simulink model "drone"  (R2020b)
settings: Solver=VariableStepAuto  StartTime=0.0  StopTime=10.0  RelTol=1e-3
settings Model: Creator=91869  LastModifiedBy=91869

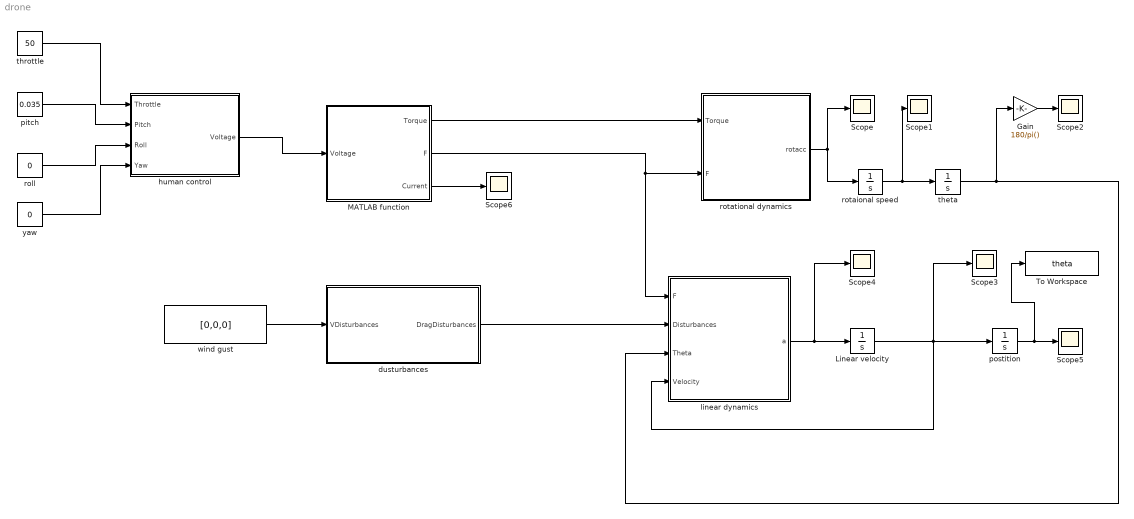
== system drone ==
  Gain : Gain  Gain=180/pi()
  Linear velocity : Integrator
  MATLAB function : MATLAB Function  TreatAsAtomicUnit=on
  Scope{,1..6} (7 alike) : Scope
  To Workspace : ToWorkspace  VariableName=theta  SampleTime=-1
      settings: Save2DSignal=2-D array (concatenate along first dimension)
  dusturbances : MATLAB Function  TreatAsAtomicUnit=on
  human control : MATLAB Function  TreatAsAtomicUnit=on
  linear dynamics : MATLAB Function  TreatAsAtomicUnit=on
  pitch : Constant  Value=0.035
  postition : Integrator
  roll : Constant  Value=0
  rotaional speed : Integrator
  rotational dynamics : MATLAB Function  TreatAsAtomicUnit=on
  theta : Integrator
  throttle : Constant  Value=50
  wind gust : Constant  Value=[0,0,0]
  yaw : Constant  Value=0
  wires:
  MATLAB function/2(F) -> linear dynamics/1(F), rotational dynamics/2(F)
  MATLAB function/1(Torque) -> rotational dynamics/1(Torque)
  rotational dynamics/1(rotacc) -> rotaional speed/1, Scope/1
  rotaional speed/1 -> Scope1/1, theta/1
  theta/1 -> Gain/1, linear dynamics/3(Theta)
  linear dynamics/1(a) -> Scope4/1, Linear velocity/1
  Linear velocity/1 -> Scope3/1, linear dynamics/4(Velocity), postition/1
  dusturbances/1(DragDisturbances) -> linear dynamics/2(Disturbances)
  wind gust/1 -> dusturbances/1(VDisturbances)
  yaw/1 -> human control/4(Yaw)
  roll/1 -> human control/3(Roll)
  pitch/1 -> human control/2(Pitch)
  throttle/1 -> human control/1(Throttle)
  human control/1(Voltage) -> MATLAB function/1(Voltage)
  postition/1 -> To Workspace/1, Scope5/1
  Gain/1 -> Scope2/1
  MATLAB function/3(Current) -> Scope6/1

== matlab function drone/rotational dynamics ==
  data: Torque input; rotacc output; F input
function rotacc = fcn(Torque,F)
Moment=[0 0 0];
rotacc=[0 0 0];
I=[0.003,0.003,0.007];
Moment(1)=(F(3)+F(4))*0.237/2-(F(1)+F(2))*0.237/2;
Moment(2)=(F(3)+F(2))*0.237/2-(F(1)+F(4))*0.237/2;
Moment(3)=Torque(4)-Torque(1)+Torque(2)-Torque(3);
for i=1:3
    rotacc(i)=Moment(i)/I(i);
end

== matlab function drone/MATLAB function ==
  data: Voltage input; Torque output; F output; Current output
function [Torque,F,Current]=fcn(Voltage)
RPM=[0 0 0 0];
Torque=[0 0 0 0];
Current=[0 0 0 0];
F=[0 0 0 0];
for i=1:4
    RPM(i)=-2.6931*Voltage(i)^3+1400*Voltage(i);
    Ct=2*10^-15*RPM(i)^3-4*10^-11*RPM(i)^2+3*10^-7*RPM(i)+0.1013;
    F(i)=Ct*1.225*(RPM(i)/60)^2*0.2^4;
    Torque(i)=4*10^-14*RPM(i)^3+8*10^-12*RPM(i)^2+3*10^-6*RPM(i);
    Current(i)=1400*Torque(i);
end

== matlab function drone/linear dynamics ==
  data: F input; a output; Disturbances input; Theta input; Velocity input
function a = fcn(F,Disturbances,Theta,Velocity)
m=0.743;
g=9.81;
A=[0.0197,0.0197,0.0512];
rho=1.225;
Cd=1;

a=[0 0 0];
Force=[0 0 0];
Fprop=[0 0 0];

Fprop(1)=sin(Theta(2))*cos(Theta(1))*(F(1)+F(2)+F(3)+F(4));
Fprop(2)=sin(Theta(1))*cos(Theta(2))*(F(1)+F(2)+F(3)+F(4));
Fprop(3)=cos(Theta(2))*cos(Theta(1))*(F(1)+F(2)+F(3)+F(4));

ThetaXY=-atan2(Fprop(1),Fprop(2));
XY2D=sqrt(Fprop(1)^2+Fprop(2)^2);

if Fprop(3)>=0
    Fprop(1)=XY2D*sin(ThetaXY+Theta(3));
    Fprop(2)=XY2D*cos(ThetaXY+Theta(3));
else
    Fprop(1)=XY2D*sin(-ThetaXY+Theta(3));
    Fprop(2)=XY2D*cos(-ThetaXY+Theta(3));
end
if Velocity(1)<0
    Force(1)=Fprop(1)-Disturbances(1)+0.5*rho*Velocity(1)^2*A(1)*Cd;
else
    Force(1)=Fprop(1)-Disturbances(1)-0.5*rho*Velocity(1)^2*A(1)*Cd;
end    
if Velocity(2)<0
    Force(2)=Fprop(2)-Disturbances(2)+0.5*rho*Velocity(2)^2*A(2)*Cd;
else
    Force(2)=Fprop(2)-Disturbances(2)-0.5*rho*Velocity(2)^2*A(2)*Cd;
end
if Velocity(3)<0
    Force(3)=Fprop(3)-Disturbances(3)+0.5*rho*Velocity(3)^2*A(3)*Cd-m*g;
else
    Force(3)=Fprop(3)-Disturbances(3)-0.5*rho*Velocity(3)^2*A(3)*Cd-m*g;
end

for i=1:3
    a(i)=Force(i)/m;
end

== matlab function drone/dusturbances ==
  data: VDisturbances input; DragDisturbances output
function DragDisturbances = fcn(VDisturbances)
A=[0.0197 0.0197 0.0197*2*1.3];
rho=1.225;
Cd=1;
DragDisturbances=[0 0 0];

for i=1:3
    if VDisturbances(i)<0
        DragDisturbances(i)=0.5*rho*VDisturbances(i)^2*A(i)*Cd;
    else    
        DragDisturbances(i)=-0.5*rho*VDisturbances(i)^2*A(i)*Cd;
    end
end

== matlab function drone/human control ==
  data: Throttle input; Voltage output; Pitch input; Roll input; Yaw input
function Voltage = fcn(Throttle,Pitch,Roll,Yaw)
Correct=0;
if (Pitch/2+Roll/2+Yaw/2)>(100-Throttle)
    Correct=(Pitch/2+Roll/2+Yaw/2)-(100-Throttle); 
end

if (Pitch/2+Roll/2+Yaw)>(Throttle-10)
    if Correct<(Pitch/2+Yaw/2+Roll/2)-(Throttle-10)
        Correct=(Pitch/2+Yaw/2+Roll/2)-(Throttle-10);
    end
end

if Correct~=0
    Pitch=Pitch-Correct/3*2;
    Roll=Roll-Correct/3*2;
    Yaw=Yaw-Correct/3*2;
end

Voltage=[(Throttle-Pitch/2-Roll/2-Yaw/2)*11.4/100 
         (Throttle-Pitch/2+Roll/2+Yaw/2)*11.4/100
         (Throttle+Pitch/2+Roll/2-Yaw/2)*11.4/100
         (Throttle+Pitch/2-Roll/2+Yaw/2)*11.4/100
                    ];
end
